simulink model "ALL_JP360_DBW_V6_5_1103"  (R2022a)
settings: Solver=FixedStepAuto  StartTime=0.0  StopTime=inf  FixedStep=0.01  RelTol=1e-3  EnableMultiTasking=on
model workspace (MAT data in the model file):
  g = 9.8
undefined symbols (not defined in the file or in its folder): canChannel, delta_v_p, IPM_Line_C0, IPM_Line_C1, IPM_Line_C2, IPM_Line_C3, M, M_p, MRR_ObjDistX, MRR_ObjDistY, MRR_ObjFusionCamID, MRR_ObjFusionSig, MRR_ObjID, MRR_ObjRelVelX, MRR_ObjRelVelY, MRR_ObjType, MRR_ObjUpdFlg, none, obj_vaild, untracktime, V, videoinput
libraries: canfdmsglib x230, canfdlib x76, slpidlib x24, simulink x18, dspstat3 x14, ctrlSharedLib x1, simulink_extras x1, imaqlib x1, realtime_pacer_lib x1, dspvision x1, visionsinks x1
(part 55 of 55)

== stateflow chart ALL_JP360_DBW_V6_5_1103/LKA_Control/Chart ==
  state ON
    state PASSIVE
      en:IPM_LineAssit_Status=1;
      state line [parallel]
        settings: executionOrder=1
        state ON
          en:y_line=y_line+1;
          du:y_line=min(y_line,51)+1;
        state OFF
          y_line=0;
        (default) -> ON.PASSIVE.line.OFF
        ON.PASSIVE.line.OFF -> ON.PASSIVE.line.ON : [Lane_status~=0]
        ON.PASSIVE.line.ON -> ON.PASSIVE.line.OFF : [Lane_status==0]
      state TorsionBarTorque [parallel] [commented out]
        state ON [commented out]
          en:y_TorsionBarTorque=y_TorsionBarTorque+1;
          du:y_TorsionBarTorque=y_TorsionBarTorque+1;
        state OFF [commented out]
          y_TorsionBarTorque=0;
        (default) -> ON.PASSIVE.TorsionBarTorque.OFF [commented out]
        ON.PASSIVE.TorsionBarTorque.OFF -> ON.PASSIVE.TorsionBarTorque.ON [commented out] : [abs(EPS_TorsionBarTorque)<1]
        ON.PASSIVE.TorsionBarTorque.ON -> ON.PASSIVE.TorsionBarTorque.OFF [commented out] : [abs(EPS_TorsionBarTorque)>=1]
    state ACTIVE
      en:IPM_LineAssit_Status=4;
      state TorsionBarTorque_jieru [parallel]
        settings: executionOrder=1
        state ON
          en:y_TorsionBarTorque_jieru=y_TorsionBarTorque_jieru+1;
          du:y_TorsionBarTorque_jieru=min(y_TorsionBarTorque_jieru,151)+1;
        state OFF
          y_TorsionBarTorque_jieru=0;
        (default) -> ON.ACTIVE.TorsionBarTorque_jieru.OFF
        ON.ACTIVE.TorsionBarTorque_jieru.OFF -> ON.ACTIVE.TorsionBarTorque_jieru.ON : [abs(EPS_TorsionBarTorque)>2]
        ON.ACTIVE.TorsionBarTorque_jieru.ON -> ON.ACTIVE.TorsionBarTorque_jieru.OFF : [abs(EPS_TorsionBarTorque)<=2]
      state line [parallel]
        settings: executionOrder=2
        state ON
          en:y_line_disappear=y_line_disappear+1;
          du:y_line_disappear=min(y_line_disappear,25)+1;
        state OFF
          y_line_disappear=0;
        (default) -> ON.ACTIVE.line.OFF
        ON.ACTIVE.line.OFF -> ON.ACTIVE.line.ON : [Lane_status==0]
        ON.ACTIVE.line.ON -> ON.ACTIVE.line.OFF : [Lane_status~=0]
    state STANDBY
      en:IPM_LineAssit_Status=1;
    (default) -> PASSIVE
    PASSIVE -> STANDBY : [BCM_DoorStsFrntLe==0x1&&BCM_DoorStsFrntRi==0x1&&BCM_DoorStsRearLe==0x1&&BCM_DoorStsRearRi==0x1&&BCM_EnginehoodSts==0x1&&SRS_SBR_Driver==0x0&&TCU_GearSelectorReq==0x5&&ABS_VehSpdLgtStatus==0x0&&ABS_VehSpdLgt>=7.1&&ABS_VehSpdLgt<=139.2&&ESP_YawRateStatus==0x0&&(abs(ESP_YawRate)<0.2)&&(Lane_status==1||Lane_status==2)&&y_line>=50&&(LaneWidth>2.6)&&(LaneCurvature<0.0033)&&(LaneChange==0)&&(ABS_AbsCtrlActv==0x0&&ESP_EspCtrlActv ==0x0)&&(abs(EPS_TorsionBarTorque)<1)&&(SWM_TurnIndicationAct~=1&&SWM_TurnIndicationAct~=2)&&SAS_SteerWheelRotSpdStatus==0x0&&(abs(SAS_SteerWheelRotSpd)<1000)&&(ESP_Master_Cylinder_Pressure_Status==0x0&&ESP_Master_Cylinder_Pressure<=10)&&abs(degre)<45]
    ACTIVE -> PASSIVE : [BCM_DoorStsFrntLe==0x2||BCM_DoorStsFrntRi==0x2||BCM_DoorStsRearLe==0x2||BCM_DoorStsRearRi==0x2||BCM_EnginehoodSts==0x2||SRS_SBR_Driver==0x2||TCU_GearSelectorReq~=0x5||(ABS_VehSpdLgtStatus==0x0&&(ABS_VehSpdLgt>143.9||ABS_VehSpdLgt<2.4))||(ESP_YawRateStatus==0x0&&abs(ESP_YawRate)>0.25)||(Lane_status==0&&y_line_disappear>24)||(LaneWidth<2.5)||LaneCurvature>0.004||LaneChange==1||(ABS_AbsCtrlActv==0x1||ESP_EspCtrlActv==0x1)||(abs(EPS_TorsionBarTorque)>2&&y_TorsionBarTorque_jieru>=150&&((EPS_TorsionBarTorque>0&&EPS_LKAResponseTorque<=0)||(EPS_TorsionBarTorque<0&&EPS_LKAResponseTorque>=0)))||((SWM_TurnIndicationAct==1||SWM_TurnIndicationAct==2)&&((acc_sta~=3&&acc_sta~=5&&acc_sta~=6)||ABS_VehSpdLgt<18))||(ESP_Master_Cylinder_Pressure_Status==0x0&&ABS_VehSpdLgt<25.9&&ESP_Master_Cylinder_Pressure>10)||(DCLC_Status==0&&Lane_status==3)||(SAS_SteerWheelRotSpdStatus==0x0&&ABS_VehSpdLgtStatus==0x0&&(abs(SAS_SteerWheelRotSpd)>1000))]
    STANDBY -> ACTIVE : [EPS_LKAControlStatus~=0x9]
  state OFF
    en:IPM_LineAssit_Status=0;
  state ERROR
    en:IPM_LineAssit_Status=5;
  (default) -> OFF
  OFF -> ON : [hasChangedFrom(LKASwitch,0)&&EPS_EPSPAMSts~=7&&EMS_IndicatedEngError==0&&MRR_HWFail==0x0&&IPM_SensorState==0x0&&ESP_EspEnableSts ==0x1]
  ON -> OFF [order 1] : [hasChangedFrom(LKASwitch,0)]
  ERROR -> OFF : [EPS_EPSPAMSts~=7&&EMS_IndicatedEngError==0&&MRR_HWFail==0x0&&IPM_SensorState==0x0&&ESP_EspEnableSts==0x1&&lka_state_sw==0]
  ON -> ERROR [order 2] : [EPS_EPSPAMSts==7||EMS_IndicatedEngError==1||MRR_HWFail==0x1||IPM_SensorState==0x4||ESP_EspEnableSts==0x0||lka_state_sw~=0]
  data: x function_input; y function_output; x function_input; y function_output; LKASwitch input int8; IPM_LineAssit_LeftVisualization input int8; IPM_LineAssit_RightVisualization input int8; SWM_TurnIndicationAct input int8; ESP_YawRateStatus input int8; ESP_YawRate input single; ABS_VehSpdLgtStatus input int8; ABS_VehSpdLgt input single; LaneCurvature input single; LaneWidth input single; LaneChange input int8; ABS_AbsCtrlActv input boolean; MRR_HWFail input boolean; IPM_SensorState input int8; lka_state_sw input int8; IPM_LineAssit_Status output int8; ESP_Master_Cylinder_Pressure input single; BCM_DoorStsFrntLe input int8; BCM_DoorStsRearRi input int8; BCM_DoorStsFrntRi input int8; BCM_DoorStsRearLe input int8; SRS_SBR_Driver input int8; BCM_EnginehoodSts input int8; TCU_GearSelectorReq input int8; EPS_TorsionBarTorque input single; EPS_LKAControlStatus input int8; ESP_EspCtrlActv input boolean; SAS_SteerWheelRotSpd input single; EPS_LKAResponseTorque input single; EPS_EPSPAMSts input int8; EMS_IndicatedEngError input boolean; ESP_EspEnableSts input boolean; SAS_SteerWheelRotSpdStatus input boolean; ESP_Master_Cylinder_Pressure_Status input boolean; y_TurnIndicatorSts local; y_TorsionBarTorque_tuoshou local; y_TorsionBarTorque_jieru local; y_TorsionBarTorque local; y_line_disappear local; y_line local; Lane_status input int8; DCLC_Status input; acc_sta input; degre input; ACC_sta input
  function y=caculate_activation(x):
    | function y=caculate_activation(x)
    |  
    | if x>=0&&x<=60
    |     y=12;
    | 
    | elseif x>60&&x<=180
    |     y=-0.1*x+18;
    | 
    | else 
    |     y=0;
    | end
    | end
  function y=caculate_deactivation(x):
    | function y=caculate_deactivation(x)
    |  
    | if x>=0&&x<=60
    |     y=10.6;
    | 
    | elseif x>60&&x<=180
    |     y=-0.08833*x+15.9;
    | 
    | else 
    |     y=0;
    | end
    | end

== matlab function ALL_JP360_DBW_V6_5_1103/LKA_Control/LKA_Cal/LKAControlerl/AngleSaftyLimitedCal ==
  data: a input single; angle_limited output single; L input single; V input single; angle input single; d_ang output single; w input single; angle_max output single
function [angle_limited,d_ang,angle_max] = fcn(a,L,V,angle, w)

angle_max = atan(a*L/V/V)*17.2*180/pi;
if angle>=0 && angle > angle_max
    angle_limited = angle_max;
elseif angle<0 && angle < -angle_max
        angle_limited = -angle_max;
else
    angle_limited = angle;
end
d_ang = 5/V/w;
end

== matlab function ALL_JP360_DBW_V6_5_1103/LKA_Control/Lane_Status/Lane_analyse ==
  data: Cl0 input single; Cl1 input; Cl2 input; Cl3 input; Cr0 input single; Cr1 input; Cr2 input; Cr3 input; Ct output single size=[1 4]; lane_status output int8; L_p input single; R_p input single; ang output single; C2 output
function [Ct,lane_status,ang,C2] = fcn(Cl0,Cl1,Cl2,Cl3,Cr0,Cr1,Cr2,Cr3,L_p,R_p)

int8 lane_status;
single Ct;

Ct = [single(0),single(0),single(0),single(0)];
if L_p > single(0.7) && L_p~=single(1) && abs(Cl0)<0.35 || R_p > single(0.7) && R_p~=single(1) && abs(Cr0)<0.35
    lane_status = int8(3);
    Ct(1) = (Cl0 + Cr0)/2;
    Ct(2) = (Cl1 + Cr1)/2;
    Ct(3) = (Cl2 + Cr2)/2;
    Ct(4) = (Cl3 + Cr3)/2;
elseif L_p > single(0.7) && R_p > single(0.7) && L_p~=single(1) && R_p~=single(1) && abs(Cl0-Cr0)>2.6 && abs(Cl0-Cr0)<5.2
    Ct(1) = (Cl0 + Cr0)/2;
    Ct(2) = (Cl1 + Cr1)/2;
    Ct(3) = (Cl2 + Cr2)/2;
    Ct(4) = (Cl3 + Cr3)/2;
    lane_status = int8(2);
elseif L_p > single(0.7) && L_p~=single(1) && abs(Cl0) < 2.6
    Ct(1) = Cl0 - single(1.7);
    Ct(2) = Cl1;
    Ct(3) = Cl2;
    Ct(4) = Cl3;
    lane_status = int8(1);
elseif R_p > single(0.7) && R_p~=single(1) && abs(Cr0) < 2.6
    Ct(1) = Cr0 + single(1.7);
    Ct(2) = Cr1;
    Ct(3) = Cr2;
    Ct(4) = Cr3;
    lane_status = int8(1);
else
    lane_status = int8(0);
    Ct(1) = (Cl0 + Cr0)/2;
    Ct(2) = (Cl1 + Cr1)/2;
    Ct(3) = (Cl2 + Cr2)/2;
    Ct(4) = (Cl3 + Cr3)/2;
end
C2 = Ct(3);
ang = abs(atan(Ct(2)))*180/pi;
end

== matlab function ALL_JP360_DBW_V6_5_1103/ACC_Control/ACC_FUNCTION/Subsystem2/ACC_model/CC_module/CalAcce ==
  data: delta_v input; y output; IC_V input
function y = fcn(delta_v, IC_V)
    if delta_v >= 2
        if IC_V < 70
            y = single(1.5);
        else
            y = single(1.3);
        end
    elseif delta_v<2 && delta_v>0.6
        y = single(0.75 * single(delta_v));
    else
        y = single(0);
%     elseif delta_v<2 && delta_v>=1.5
%         y = 1.2;
%     elseif delta_v<1.5 && delta_v>=0.5
%         y = 0.8;
%     else
%         y =0;
    end
end

== matlab function ALL_JP360_DBW_V6_5_1103/CIPV1/Lane Line Construction1/Embedded MATLAB Function5 ==
  data: judge output; IPM_Line_type input; IPM_Line_Existence_Probability input; IPM_Line_C0 input; line_data output; IPM_Line_C1 input; IPM_Line_C2 input; IPM_Line_C3 input; judge_cover_line_left input; judge_cover_line_right input
function [judge, line_data] = line_fun(IPM_Line_type, IPM_Line_Existence_Probability, IPM_Line_C0, IPM_Line_C1, IPM_Line_C2, IPM_Line_C3, judge_cover_line_left, judge_cover_line_right)
judge = 0;
% Judge whether it is a road edge
if IPM_Line_type == 2
    line_data = single([0, 0, 0, 0]);
else
    if IPM_Line_Existence_Probability >= 50 && judge_cover_line_left==0 && judge_cover_line_right==0
        line_data = single([IPM_Line_C0, IPM_Line_C1, IPM_Line_C2, IPM_Line_C3]);
        judge = 1;
    else
        line_data = single([0,0,0,0]);
        judge = 0;
    end
end
end

== stateflow chart ALL_JP360_DBW_V6_5_1103/ACC_Control/ACC_FUNCTION/Subsystem2/Limit/Chart1 ==
  state a
    state OFF
      trottle=0;
      brake=dec;
    state OFF1
      trottle=acc;
      brake=0;
    state ON
      trottle=t;
      brake=0;
    a -> (junction 1)
    (junction 1) -> OFF1 [order 3]
    (default) -> (junction 1)
    (junction 1) -> OFF [order 2] : [abs(dec)>brake_kt]
    (junction 1) -> ON [order 1] : [dec~=0&&abs(dec)<=brake_kt]
  (default) -> a
  data: trottle output single; acc input; brake_kt input; dec input; brake output single; t input

== stateflow chart ALL_JP360_DBW_V6_5_1103/ACC_Control/ACC_FUNCTION/Subsystem2/Limit/acceleration_throttle——PID/Out_PID/30-1/Chart8 ==
  settings: executeAtInitialization=1
  state s
    state else
      P=0;
      I=0;
      D=0;
      N=0;
    state V30_40
      P=110;
      I=3;
      D=0;
      N=100;
    state V41_50
      P=120;
      I=5;
      D=0;
      N=100;
    state V51_60
      P=130;
      I=5;
      D=0;
      N=100;
    state V61_70
      P=135;
      I=5;
      D=0;
      N=100;
    state V71_80
      P=140;
      I=5;
      D=0;
      N=100;
    state V81_90
      P=135;
      I=5.5;
      D=0;
      N=100;
    state V91_100
      P=130;
      I=5.8;
      D=0;
      N=100;
    state V101_110
      P=130;
      I=6;
      D=0;
      N=100;
    state V111_120
      P=130;
      I=6.5;
      D=0;
      N=100;
    state V121_130
      P=135;
      I=6.5;
      D=0;
      N=100;
    state V131_140
      P=135;
      I=6.8;
      D=0;
      N=100;
    state V141_150
      P=135;
      I=7;
      D=0;
      N=100;
    s -> (junction 54)
    (default) -> else
    (junction 54) -> V111_120 [order 9] : [speed>=111&&speed<=120]
    (junction 54) -> V30_40 [order 1] : [speed>=30&&speed<=40]
    (junction 54) -> V101_110 [order 8] : [speed>=101&&speed<=110]
    (junction 54) -> V141_150 [order 12] : [speed>=141&&speed<=150]
    (junction 54) -> V131_140 [order 11] : [speed>=131&&speed<=140]
    (junction 54) -> V81_90 [order 6] : [speed>=81&&speed<=90]
    (junction 54) -> V51_60 [order 3] : [speed>=51&&speed<=60]
    (junction 54) -> V121_130 [order 10] : [speed>=121&&speed<=130]
    (junction 54) -> V61_70 [order 4] : [speed>=61&&speed<=70]
    (junction 54) -> V71_80 [order 5] : [speed>=71&&speed<=80]
    (junction 54) -> V91_100 [order 7] : [speed>=91&&speed<=100]
    (junction 54) -> V41_50 [order 2] : [speed>=41&&speed<=50]
  (default) -> s
  data: P output uint8; speed input; I output single; D output single; N output int8
